simulink model "Tutorial_Simulink_2"  (R2023b)
settings: Solver=VariableStepAuto  StartTime=0.0  StopTime=10.0  RelTol=1e-3
settings Model: Creator=admin  LastModifiedBy=admin

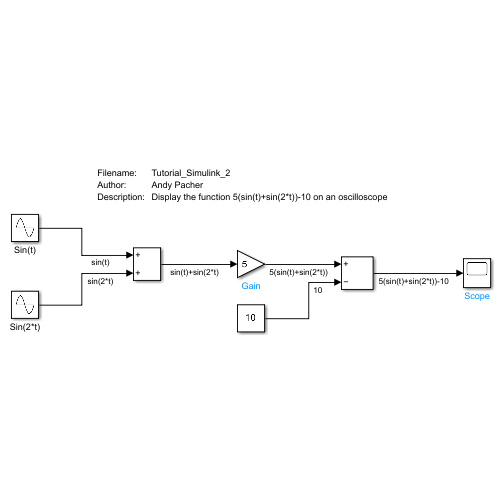
[thumbnail: Simulink's stored preview of the top-level diagram]
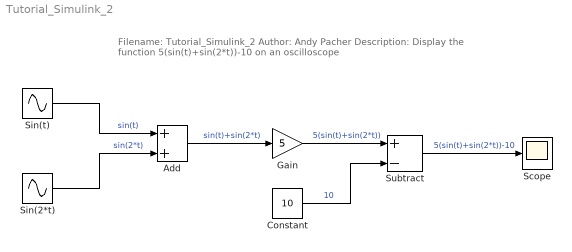
== system Tutorial_Simulink_2 ==
  note: Filename:	Tutorial_Simulink_2
      | Author:		Andy Pacher
      | Description:	Display the function 5(sin(t)+sin(2*t))-10 on an oscilloscope
  Add : Sum
  Constant : Constant  Value=10
  Gain : Gain  Gain=5
  Scope : Scope
  Sin(2*t) : Sin  Frequency=2  SampleTime=0
  Sin(t) : Sin  SampleTime=0
  Subtract : Sum  Inputs=+-
  wires:
  Gain/1 -> Subtract/1  "5(sin(t)+sin(2*t))"
  Constant/1 -> Subtract/2  "10"
  Add/1 -> Gain/1  "sin(t)+sin(2*t)"
  Sin(t)/1 -> Add/1  "sin(t)"
  Sin(2*t)/1 -> Add/2  "sin(2*t)"
  Subtract/1 -> Scope/1  "5(sin(t)+sin(2*t))-10"
